simulink model "Kalman_Filter_sim_model"  (R2020a)
settings: Solver=FixedStepAuto  StartTime=0.0  StopTime=t(end)  FixedStep=Ts  RelTol=1e-3
values from neighbouring files (symbols this model uses):
  A = Model.A    [GPB1_estimation.m]    (also in GPB1_estimation_BT.m; GPB2_estimation.m)
  B = Model.B    [GPB1_estimation_BT.m]
  C = Model.C    [GPB1_estimation.m]    (also in GPB1_estimation_BT.m; GPB2_estimation.m; MKFObserverA.m = obj.filters{f}.C)
  N = size(Model.A{1},1)    [GPB1_estimation.m]    (also in GPB1_estimation_BT.m = size(Model.A,1); GPB2_estimation.m = size(Model.A{1}, 1))
  R = Model.R    [GPB1_estimation.m]    (also in GPB1_estimation_BT.m; GPB2_estimation.m; MEKF_observer_RODD.m = repmat({R}, 1, nj))
  x0 = zeros(n, 1)    [AbstractLinearFilter.m]    (also in KalmanFilter.m; KalmanFilterSS_sfunc.m = obs.xkp1_est; MEKF_observer_RODD.m; MKFObserver.m)
undefined symbols (not defined in the file or in its folder): Discrete, Time, Ts
libraries: ctrlSharedLib x1
settings Model: Creator=Andre  LastModifiedBy=billtubbs
settings DataIOCC: ReturnWorkspaceOutputs=off
settings DebuggingCC: ArithmeticOperatorsInVariantConditions=warning
settings SFSimCC: SimUseLocalCustomCode=off  CustomCodeUndefinedFunction=UseInterfaceOnly
settings RTWCC: RTWUseLocalCustomCode=off

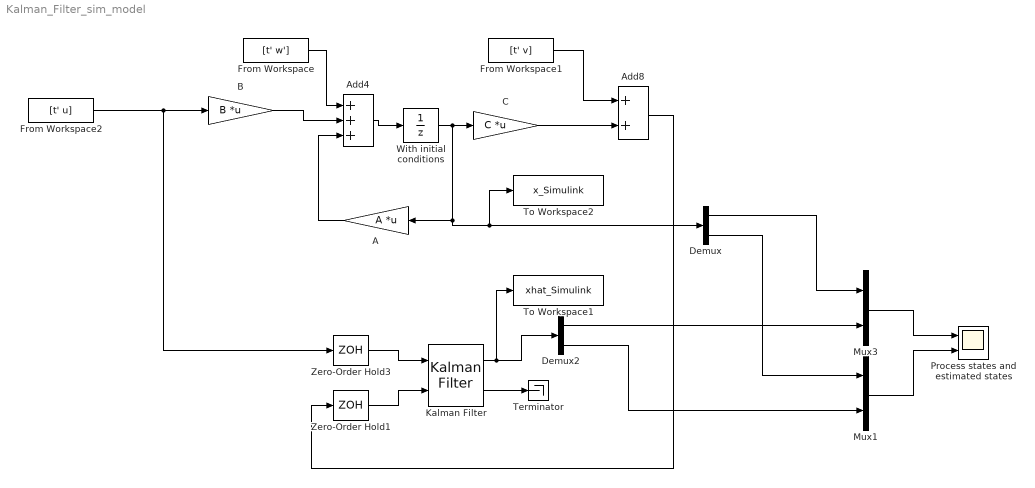
== system Kalman_Filter_sim_model ==
  A : Gain  Gain=A  Multiplication=Matrix(K*u)
  Add4 : Sum  Inputs=+++
  Add8 : Sum
  B : Gain  Gain=B  Multiplication=Matrix(K*u)
  C : Gain  Gain=C  Multiplication=Matrix(K*u)
  Demux : Demux  Outputs=2
  Demux2 : Demux  Outputs=2
  From Workspace : FromWorkspace  VariableName=[t' w']
  From Workspace1 : FromWorkspace  VariableName=[t' v]
  From Workspace2 : FromWorkspace  VariableName=[t' u]
  Kalman Filter : ctrlSharedLib/Kalman Filter  TimeDomain=Discrete-Time  UseCurrentEstimator=off  ModelSource=LTI State-Space Variable  ModelSourceVariable=G  A=0.95  B=1  C=1  D=0  NumberOfStates=1  NumberOfInputs=1  NumberOfOutputs=1  InitialEstimateSource=Dialog  X0=0  P0=10  UseK=off  UseGH=on  NumberOfProcessNoiseInputs=1  G=Gkf  TimeInvariantG=on  H=Hkf  TimeInvariantH=on  Q=Q  TimeInvariantQ=on  R=R  TimeInvariantR=on  N=N  TimeInvariantN=on  AddInputPort=on  AddEnablePort=off  OutputEstimatedY=on  OutputP=off  Ts=-1
  Mux1 : Mux  Inputs=2
  Mux3 : Mux  Inputs=2
  Process states and estimated states : Scope  NumInputPorts=2
  Terminator : Terminator
  To Workspace1 : ToWorkspace  VariableName=xhat_Simulink  SaveFormat=Timeseries  SampleTime=-1
  To Workspace2 : ToWorkspace  VariableName=x_Simulink  SaveFormat=Timeseries  SampleTime=-1
  With initial conditions : UnitDelay  InitialCondition=x0  SampleTime=Ts  HasFrameUpgradeWarning=on
  Zero-Order Hold1 : ZeroOrderHold  SampleTime=Ts
  Zero-Order Hold3 : ZeroOrderHold  SampleTime=Ts
  wires:
  A/1 -> Add4/3
  Mux1/1 -> Process states and estimated states/2
  Demux/1 -> Mux3/1
  Demux/2 -> Mux1/1
  Add4/1 -> With initial conditions/1
  From Workspace/1 -> Add4/1
  B/1 -> Add4/2
  With initial conditions/1 -> C/1, To Workspace2/1, Demux/1, A/1
  C/1 -> Add8/2
  From Workspace1/1 -> Add8/1
  Kalman Filter/1 -> To Workspace1/1, Demux2/1
  Demux2/1 -> Mux3/2
  Demux2/2 -> Mux1/2
  Add8/1 -> Zero-Order Hold1/1
  From Workspace2/1 -> Zero-Order Hold3/1, B/1
  Zero-Order Hold3/1 -> Kalman Filter/1
  Zero-Order Hold1/1 -> Kalman Filter/2
  Mux3/1 -> Process states and estimated states/1
  Kalman Filter/2 -> Terminator/1
